simulink model "TD2_Exercise_12"  (R2021a)
settings: Solver=VariableStepAuto  StartTime=0.0  StopTime=0.01666666667  RelTol=1e-3
libraries: spsMeanLib x2, spsRMSLib x2, spsVoltageMeasurementLib x2, spsACVoltageSourceLib x1, spsDCVoltageSourceLib x1, spsCurrentMeasurementLib x1, spsSeriesRLCBranchLib x1, spsThyristorLib x1, spspowerguiLib x1
settings Model: Creator=lundy  LastModifiedBy=lundy

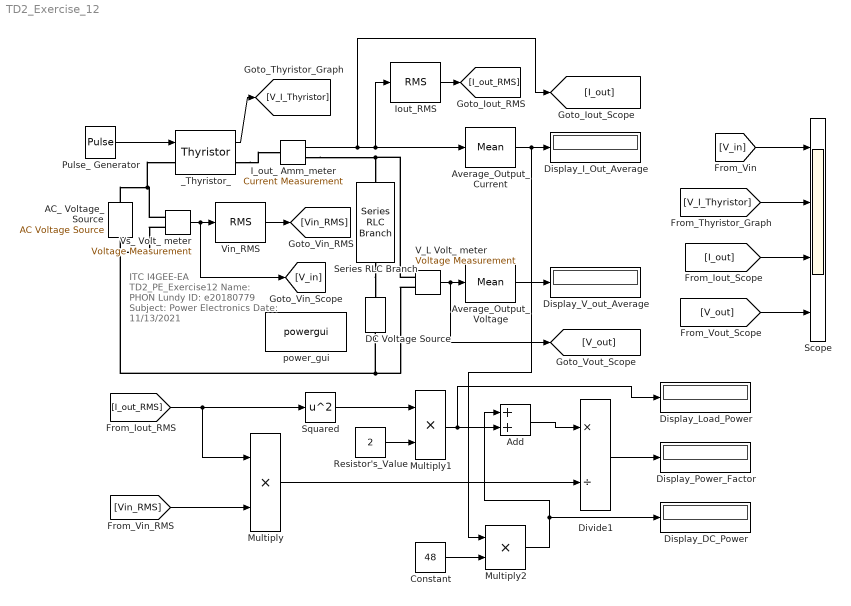
== system TD2_Exercise_12 ==
  note: ITC I4GEE-EA
      | TD2_PE_Exercise12
      | Name:     PHON Lundy
      | ID:       	 e20180779
      | Subject:  Power Electronics
      | Date:      11/13/2021
  AC_ Voltage_ Source : spsACVoltageSourceLib/AC Voltage Source  Amplitude=120*sqrt(2)  Phase=0  Frequency=60  SampleTime=0  Measurements=None  BusType=swing  Pref=10e3  Qref=0  Qmin=-inf  Qmax=+inf
  Add : Sum
  Average_Output_ Current : spsMeanLib/Mean  Freq=60  Vinit=240  Ts=0
  Average_Output_ Voltage : spsMeanLib/Mean  Freq=60  Vinit=240  Ts=0
  Constant : Constant  Value=48
  DC Voltage Source : spsDCVoltageSourceLib/DC Voltage Source  Amplitude=48  Measurements=None
  Display_DC_Power : Display
  Display_I_Out_Average : Display
  Display_Load_Power : Display
  Display_Power_Factor : Display
  Display_V_out_Average : Display
  Divide1 : Product  Inputs=*/
  I_out_ Amm_meter : spsCurrentMeasurementLib/Current Measurement  PhasorSimulation=off  OutputType=Complex  PSBequivalent=0
  Iout_RMS : spsRMSLib/RMS  TrueRMS=on  Freq=60  RMSInit=240  Ts=0
  Multiply : Product
  Multiply1 : Product
  Multiply2 : Product
  Pulse_ Generator : DiscretePulseGenerator  PulseType=Time based  Period=1/60  PulseWidth=50  PhaseDelay=0.8726/(pi*2*60)
  Resistor's_Value : Constant  Value=2
  Scope : Scope  NumInputPorts=4
  Series RLC Branch : spsSeriesRLCBranchLib/Series RLC Branch  LConnTagsString=__new0  RConnTagsString=__new0  BranchType=RL  Resistance=2  Inductance=0.075  SetiL0=off  InitialCurrent=0  Capacitance=1e-6  Setx0=off  InitialVoltage=0  Measurements=None
  Squared : Math  Operator=square  SaturateOnIntegerOverflow=on
  V_L Volt_ meter : spsVoltageMeasurementLib/Voltage Measurement  PhasorSimulation=off  OutputType=Complex  PSBequivalent=0
  Vin_RMS : spsRMSLib/RMS  TrueRMS=on  Freq=60  RMSInit=240  Ts=0
  Vs_ Volt_ meter : spsVoltageMeasurementLib/Voltage Measurement  PhasorSimulation=off  OutputType=Complex  PSBequivalent=0
  _Thyristor_ : spsThyristorLib/Thyristor  Ron=0.001  Lon=0  Vf=0.8  IC=0  Rs=inf  Cs=inf  Measurements=on
  power_gui : spspowerguiLib/powergui  Priority=1  SimulationMode=Continuous  SampleTime=50e-6  frequency=60  Iterations=50  frequencyindice=60  Pbase=100e6  ErrMax=1e-4  UnitsV=kV  UnitsW=MW  buscounter=0  FunctionMessages=off  echomessages=off  EnableUseOfTLC=off  CurrentSourceSwitches=off  DisableSnubberDevices=off  DisableRonSwitches=off  DisableVfSwitches=off  DisplayEquations=off  AutomaticDiscreteSolvers=off  SolverType=Tustin/Backward Euler (TBE)  Interpol=off  ExternalGateDelay=off  methode=off  Ts=100  x0status=blocks  SPID=on  SwTol=0  HookPort=off  NonlinearTolerance=1e-4  nMaxIteration=100  ContinueOnMaxIteration=off  RestoreLinks=warning  ResistiveCurrentMeasurement=off  Frange=[0:2:500]  Ylog=off  Xlog=on  ShowGrid=off  save=off  variable=ZData  structure=0  ZoomFFT=off  StartTime=0.0  cycles=1  DisplayStyle=1  fundamental=60  FreqAxis=off  MaxFrequency=1000  frequencyindicesteady=1  RmsSteady=1  display=off
  wires:
  Pulse_ Generator/1 -> _Thyristor_/1
  V_L Volt_ meter/1 -> [V_out], Average_Output_ Voltage/1
  Average_Output_ Voltage/1 -> Display_V_out_Average/1
  _Thyristor_/1 -> [V_I_Thyristor]
  Vs_ Volt_ meter/1 -> [V_in], Vin_RMS/1
  Vin_RMS/1 -> [Vin_RMS]
  Iout_RMS/1 -> [I_out_RMS]
  [I_out_RMS] -> Multiply/1, Squared/1
  Multiply/1 -> Divide1/2
  Divide1/1 -> Display_Power_Factor/1
  [V_in] -> Scope/1
  [I_out] -> Scope/3
  [V_I_Thyristor] -> Scope/2
  [V_out] -> Scope/4
  I_out_ Amm_meter/1 -> Average_Output_ Current/1, Iout_RMS/1, [I_out]
  [Vin_RMS] -> Multiply/2
  Squared/1 -> Multiply1/1
  Resistor's_Value/1 -> Multiply1/2
  Multiply1/1 -> Display_Load_Power/1, Add/2
  Constant/1 -> Multiply2/2
  Average_Output_ Current/1 -> Multiply2/1, Display_I_Out_Average/1
  Multiply2/1 -> Display_DC_Power/1, Add/1
  Add/1 -> Divide1/1
  connections:
  Series RLC Branch/RConn1 -- DC Voltage Source/RConn1
  I_out_ Amm_meter/RConn1 -- Series RLC Branch/LConn1 -- V_L Volt_ meter/LConn1
  _Thyristor_/RConn1 -- I_out_ Amm_meter/LConn1
  AC_ Voltage_ Source/RConn1 -- _Thyristor_/LConn1 -- Vs_ Volt_ meter/LConn1
  V_L Volt_ meter/LConn2 -- DC Voltage Source/LConn1 -- AC_ Voltage_ Source/LConn1 -- Vs_ Volt_ meter/LConn2
